simulink model "Elevator_Incorrect_abiadura_Ur1_12"  (R2024a)
settings: Solver=VariableStepAuto  StartTime=0.0  StopTime=120  RelTol=1e-3
undefined symbols (not defined in the file or in its folder): sigbuilder_block
settings Model: Creator=mugarte  LastModifiedBy=airshad
settings RTWCC: GPUComputeCapability=3.5

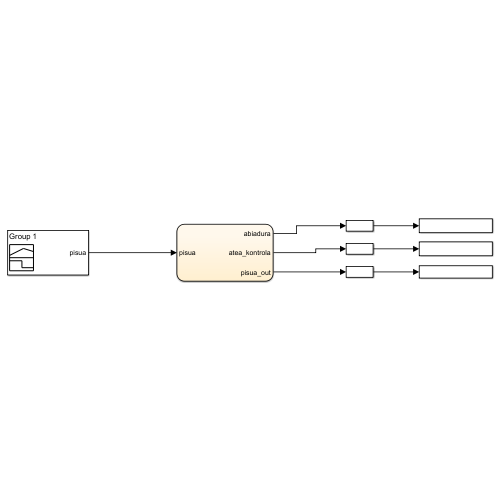
[thumbnail: Simulink's stored preview of the top-level diagram]
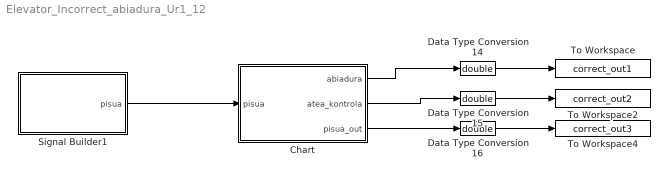
== system Elevator_Incorrect_abiadura_Ur1_12 ==
  Chart : Stateflow chart  TreatAsAtomicUnit=on
  Data Type Conversion14 : DataTypeConversion  OutDataTypeStr=double  SaturateOnIntegerOverflow=off  RndMeth=Floor
  Data Type Conversion15 : DataTypeConversion  OutDataTypeStr=double  SaturateOnIntegerOverflow=off  RndMeth=Floor
  Data Type Conversion16 : DataTypeConversion  OutDataTypeStr=double  SaturateOnIntegerOverflow=off  RndMeth=Floor
  Signal Builder1 : Subsystem  Tag=STV Subsys  LoadFcn=sigbuilder_block('load');  StartFcn=sigbuilder_block('start');  StopFcn=sigbuilder_block('stop');  ClipboardFcn=sigbuilder_block('clipboard');  mask(Sigbuilder block){tuvar=[0:10]}
      mask help: Simulink:masks:SigbuilderBlock_MD
      mask init:
      | if ~strcmp(get_param(bdroot(gcbh),'SimulationStatus'),'stopped') tuvar = sigbuilder_block('maskInit'); end
      settings: CopyFcn=sigbuilder_block('copy');  DeleteFcn=sigbuilder_block('delete');  ModelCloseFcn=sigbuilder_block('modelClose');  PreSaveFcn=sigbuilder_block('preSave');  PauseFcn=sigbuilder_block('pause');  ContinueFcn=sigbuilder_block('continue');  NameChangeFcn=sigbuilder_block('namechange');  OpenFcn=sigbuilder_block('open',[883.5 210.75 550.5 240.75 ]);  CloseFcn=sigbuilder_block('close');
      mask Display: plot(0, 0, 100, 100,[2, 2, 32, 32, 2], [68, 8, 8, 68, 68],[32, 2], [38, 38], [32, 19, 2],[53, 60, 44], [32, 17, 17, 2],[16, 16, 31, 31]);txt = getActiveGroup(gcbh);text(2, 100, txt,'verticalAlignment', 'top');
  To Workspace : ToWorkspace  VariableName=correct_out1  SaveFormat=Timeseries  SampleTime=-1
  To Workspace2 : ToWorkspace  VariableName=correct_out2  SaveFormat=Timeseries  SampleTime=-1
  To Workspace4 : ToWorkspace  VariableName=correct_out3  SaveFormat=Timeseries  SampleTime=-1
  wires:
  Signal Builder1/1(pisua) -> Chart/1(pisua)
  Data Type Conversion15/1 -> To Workspace2/1
  Chart/3(pisua_out) -> Data Type Conversion16/1
  Data Type Conversion14/1 -> To Workspace/1
  Data Type Conversion16/1 -> To Workspace4/1
  Chart/1(abiadura) -> Data Type Conversion14/1
  Chart/2(atea_kontrola) -> Data Type Conversion15/1

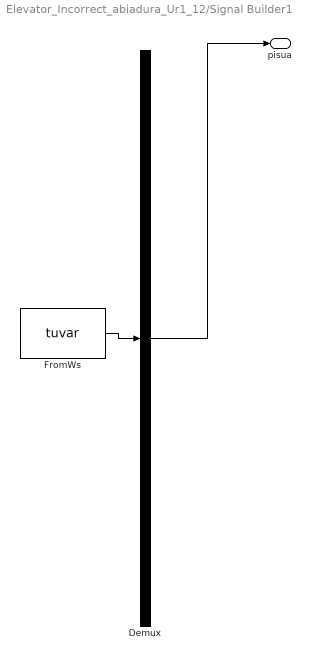
== system Elevator_Incorrect_abiadura_Ur1_12/Signal Builder1 ==
  Demux : Demux  Tag=STV Demux  Outputs=1
      settings: DisplayOption=none
  FromWs : FromWorkspace  Tag=STV FromWs  VariableName=tuvar
      SigBuilderData=|
      | common.afterFinalStr = 'Extrapolate'
      | common.sampleTime = 0
      | dataSet(1).timeRange = [0 120]
      | dataSet(1).name = 'Group 1'
      | dataSet(2).timeRange = [0 120]
      | dataSet(2).name = 'Group 2'
      | dataSet(3).timeRange = [0 120]
      | dataSet(3).name = 'Group 3'
      | sbobj.Groups(1).Name = 'Group 1'
      | sbobj.Groups(1).Signals.Name = 'pisua'
      | sbobj.Groups(1).Signals.XData = [0 120]
      | sbobj.Groups(1).Signals.YData = [5 5]
      | sbobj.Groups(1).TimeRange = [0 120]
      | sbobj.Groups(2).Name = 'Group 2'
      | sbobj.Groups(2).Signals.Name = 'pisua'
      | sbobj.Groups(2).Signals.XData = [0 120]
      | sbobj.Groups(2).Signals.YData = [-2 -2]
      | sbobj.Groups(2).TimeRange = [0 120]
      | sbobj.Groups(3).Name = 'Group 3'
      | sbobj.Groups(3).Signals.Name = 'pisua'
      | sbobj.Groups(3).Signals.XData = [0 120]
      | sbobj.Groups(3).Signals.YData = [0 0]
      | sbobj.Groups(3).TimeRange = [0 120]
  pisua : Outport  Tag=STV Outport
  wires:
  FromWs/1 -> Demux/1
  Demux/1 -> pisua/1

== stateflow chart Elevator_Incorrect_abiadura_Ur1_12/Chart ==
  state Geldirik
    entry:
    atea_kontrola=0;
    abiadura=0;
    pisua_out=oraingoPisua;
  state ateak_ixten
    entry:
    atea_kontrola=-1;
    exit:
    atea_kontrola=0;
  state jaisten
    entry:
    abiadura=10;
    pisua_out=oraingoPisua;
  state igotzen
    entry:
    pisua_out=oraingoPisua;
  state ateak_irekitzen
    entry:
    abiadura=0;
    atea_kontrola=1;
  (default) -> Geldirik : {oraingoPisua=0;}
  ateak_irekitzen -> Geldirik : after(3,sec)
  Geldirik -> ateak_ixten : [pisua~=oraingoPisua]
  ateak_ixten -> (junction 33) : [after(3,sec)]
  (junction 33) -> (junction 39) [order 2] : [pisua<oraingoPisua]
  (junction 33) -> (junction 36) [order 1] : [pisua>oraingoPisua]
  (junction 39) -> jaisten
  (junction 36) -> igotzen : [pisua > 0]
  jaisten -> jaisten [order 2] : after(5, sec){oraingoPisua = oraingoPisua - 1;}
  igotzen -> igotzen [order 2] : after(10, sec){oraingoPisua = oraingoPisua + 1;
      | }
  jaisten -> ateak_irekitzen [order 1] : [pisua==oraingoPisua]
  igotzen -> ateak_irekitzen [order 1] : [pisua==oraingoPisua]
  data: pisua input; abiadura output; atea_kontrola output; pisua_out output; oraingoPisua local
